simulink model "SS_F16_Block_lo"  (Simulink 9.2)
settings: Solver=ode5  StartTime=0.0  StopTime=5  FixedStep=deltaT  RelTol=1e-3  EnableMultiTasking=on
values from neighbouring files (symbols this model uses):
  A = state_space.A_lo    [open_loop_response.m]    (also in runLINF16sim.m = A_lo; terrain_following_model.m)
  B = state_space.B_lo    [open_loop_response.m]    (also in runLINF16sim.m = B_lo; terrain_following_model.m)
  C = state_space.C_lo    [open_loop_response.m]    (also in runLINF16sim.m = C_lo; terrain_following_model.m)
  D = state_space.D_lo    [open_loop_response.m]    (also in runLINF16sim.m = D_lo; terrain_following_model.m)
  thrust = 5000    [FindF16Dynamics.m]    (also in normal_response_wrt_acc_pos.m = 0; runF16Sim.m; runLINF16sim.m = 0; sim_F16_lo.m = 0)
  trim_control = trim_control_lo    [runLINF16sim.m]    (also in trim_F16.m = [UX(2);UX(4);UX(5)]; trim_steady_state.m = [UX(2);UX(4);UX(5)])
  trim_state = xu_lo    [runLINF16sim.m]    (also in trim_F16.m = xu(1:12); trim_steady_state.m = xu(1:12))
  trim_thrust = trim_thrust_lo    [runLINF16sim.m]    (also in trim_F16.m = UX(1); trim_steady_state.m = UX(1))
settings Model: Creator=russ1110  LastModifiedBy=lorenzoterenzi  ExtModeAutoUpdateStatusClock=off
settings DataIOCC: SignalLoggingName=sigsOut
settings OptimizationCC: BooleanDataType=off  LifeSpan=auto
settings DebuggingCC: SaveWithParameterizedLinksMsg=none  SignalResolutionControl=TryResolveAllWithWarning  MultiTaskDSMMsg=warning  MultiTaskCondExecSysMsg=none  FcnCallInpInsideContextMsg=error  StateNameClashWarn=none  SFUnexpectedBacktrackingDiag=error  SFNoUnconditionalDefaultTransitionDiag=error  SFExecutionAtInitializationDiag=warning
settings HardwareCC: TargetUnknown=on
settings SFSimCC: SimUseLocalCustomCode=on
settings RTWCC: RTWUseLocalCustomCode=on
settings CodeAppCC: StateflowObjectComments=off
settings GRTTargetCC: TargetLangStandard=C99 (ISO)  GeneratePreprocessorConditionals=Use local settings
settings ConfigComp: CovExternalEMLEnable=on

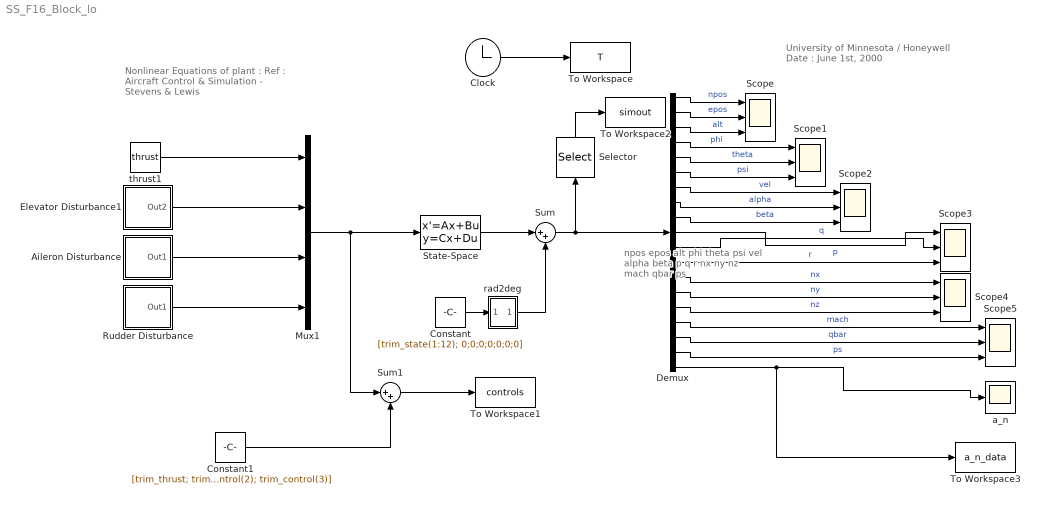
== system SS_F16_Block_lo ==
  note: npos
      | epos
      | alt
      | phi
      | theta
      | psi
      | vel
      | alpha
      | beta
      | p
      | q
      | r
      | nx
      | ny
      | nz
      | mach
      | qbar
      | ps
  note: University of Minnesota / Honeywell
      | Date : June 1st, 2000
  note: Nonlinear Equations of plant :
      | Ref : Aircraft Control & Simulation
      | - Stevens & Lewis
  Aileron Disturbance : Subsystem
  Clock : Clock
      settings: Decimation=50
  Constant : Constant  Value=[trim_state(1:12); 0;0;0;0;0;0;0]
  Constant1 : Constant  Value=[trim_thrust; trim_control(1); trim_control(2); trim_control(3)]
  Demux : Demux  Outputs=19
  Elevator Disturbance1 : Subsystem
  Mux1 : Mux
  Rudder Disturbance : Subsystem
  Scope{,1..5} (6 alike) : Scope  NumInputPorts=3
  Selector : Selector  InputPortWidth=19  IndexOptions=Index vector (dialog)  Indices=[1:18]  OutputSizes=1
  State-Space : StateSpace  A=A  B=B  C=C  D=D  InitialCondition=0
  Sum : Sum  Inputs=|++  SaturateOnIntegerOverflow=on  InputSameDT=on  OutDataTypeStr=Inherit: Same as first input
  Sum1 : Sum  Inputs=|++  SaturateOnIntegerOverflow=on  InputSameDT=on  OutDataTypeStr=Inherit: Same as first input
  To Workspace : ToWorkspace  VariableName=T  SampleTime=-1
      settings: Decimation=100
  To Workspace1 : ToWorkspace  VariableName=controls  SampleTime=-1
      settings: Decimation=100
  To Workspace2 : ToWorkspace  VariableName=simout  SampleTime=-1
      settings: Decimation=100
  To Workspace3 : ToWorkspace  VariableName=a_n_data  SaveFormat=Timeseries  SampleTime=-1
  "a_n " : Scope
  rad2deg : Subsystem
  thrust1 : Constant  Value=thrust  VectorParams1D=off
  wires:
  Clock/1 -> To Workspace/1
  Demux/1 -> Scope/1  "npos"
  Demux/2 -> Scope/2  "epos"
  Demux/3 -> Scope/3  "alt"
  Demux/5 -> Scope1/2  "theta"
  Demux/6 -> Scope1/3  "psi"
  Demux/7 -> Scope2/1  "vel"
  Demux/8 -> Scope2/2  "alpha"
  Demux/9 -> Scope2/3  "beta"
  Demux/10 -> Scope3/1  "p"
  Demux/11 -> Scope3/2  "q"
  Demux/12 -> Scope3/3  "r"
  Demux/13 -> Scope4/1  "nx"
  Demux/14 -> Scope4/2  "ny"
  Demux/15 -> Scope4/3  "nz"
  Demux/4 -> Scope1/1  "phi"
  Demux/16 -> Scope5/1  "mach"
  Demux/17 -> Scope5/2  "qbar"
  Demux/18 -> Scope5/3  "ps"
  State-Space/1 -> Sum/1
  Sum/1 -> Demux/1, Selector/1
  thrust1/1 -> Mux1/1
  Aileron Disturbance/1(Out1) -> Mux1/3
  Rudder Disturbance/1(Out1) -> Mux1/4
  Constant1/1 -> Sum1/2
  Mux1/1 -> State-Space/1, Sum1/1
  Sum1/1 -> To Workspace1/1
  rad2deg/1(Out1) -> Sum/2
  Demux/19 -> To Workspace3/1, "a_n "/1
  Constant/1 -> rad2deg/1(In1)
  Selector/1 -> To Workspace2/1
  Elevator Disturbance1/1(Out2) -> Mux1/2

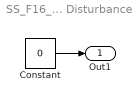
== system SS_F16_Block_lo/Aileron Disturbance ==
  Constant : Constant  Value=0
  Out1 : Outport
  wires:
  Constant/1 -> Out1/1

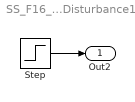
== system SS_F16_Block_lo/Elevator Disturbance1 ==
  Step : Step  Time=0  After=-1  SampleTime=0
  Out2 : Outport
  wires:
  Step/1 -> Out2/1

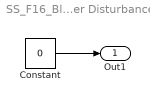
== system SS_F16_Block_lo/Rudder Disturbance ==
  Constant : Constant  Value=0
  Out1 : Outport
  wires:
  Constant/1 -> Out1/1

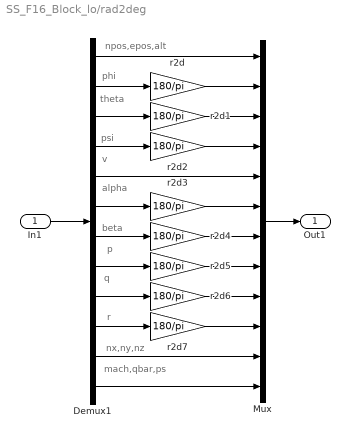
== system SS_F16_Block_lo/rad2deg ==
  note: npos,epos,alt
  note: phi
  note: theta
  note: psi
  note: v
  note: alpha
  note: beta
  note: p
  note: q
  note: r
  note: nx,ny,nz
  note: mach,qbar,ps
  In1 : Inport
  Demux1 : Demux  Outputs=[3 1 1 1 1 1 1 1 1 1 3 4]
  Mux : Mux  Inputs=[3 1 1 1 1 1 1 1 1 1 3 4]
  r2d{,1..7} (8 alike) : Gain  Gain=180/pi  SaturateOnIntegerOverflow=on  OutDataTypeStr=Inherit: Same as input  ParamDataTypeStr=Inherit: Same as input
  Out1 : Outport
  wires:
  In1/1 -> Demux1/1
  Demux1/2 -> r2d/1
  Demux1/3 -> r2d1/1
  Demux1/4 -> r2d2/1
  Demux1/1 -> Mux/1
  Demux1/5 -> Mux/5
  r2d2/1 -> Mux/4
  r2d1/1 -> Mux/3
  r2d/1 -> Mux/2
  Demux1/6 -> r2d3/1
  Demux1/7 -> r2d4/1
  Demux1/8 -> r2d5/1
  Demux1/9 -> r2d6/1
  Demux1/10 -> r2d7/1
  r2d3/1 -> Mux/6
  r2d4/1 -> Mux/7
  r2d5/1 -> Mux/8
  r2d6/1 -> Mux/9
  r2d7/1 -> Mux/10
  Mux/1 -> Out1/1
  Demux1/11 -> Mux/11
  Demux1/12 -> Mux/12
